simulink model "playground"  (R2024a)
settings: Solver=ode45  StartTime=0.0  StopTime=10.0  FixedStep=0.001  RelTol=1e-3
values from neighbouring files (symbols this model uses):
  a_r = 1.14 * 10^(-7)    (= 1.14e-07)    [start.m]    (also in startEnglPaper.m = 0.033; startReduced.m)
  a_rS = b    (= 0.033)    [startEnglPaper.m]
  A_x = 0.25    [playgrounMat.m]    (also in start.m; startEnglPaper.m; startReduced.m)
  A_y = 0.25    [playgrounMat.m]    (also in start.m; startEnglPaper.m; startReduced.m)
  A_z = 0.25    [playgrounMat.m]    (also in start.m; startEnglPaper.m; startReduced.m)
  b = 1.14 * 10^(-7)    (= 1.14e-07)    [start.m]    (also in startEnglPaper.m = 0.033; startReduced.m)
  g = 9.81    [playgrounMat.m]    (also in start.m; startEnglPaper.m; startReduced.m)
  gamma_d = pi/3    (= 1.0471975512)    [start.m]    (also in startReduced.m)
  I_r = 5.38 * 10 ^ (-5)    (= 5.38e-05)    [start.m]    (also in startEnglPaper.m = 3.38e-05; startReduced.m)
  I_x = 0.0151    [start.m]    (also in startEnglPaper.m = 0.004856; startReduced.m)
  I_y = 0.253    [start.m]    (also in startEnglPaper.m = 0.004856; startReduced.m)
  I_z = 0.0151    [start.m]    (also in startEnglPaper.m = 0.008801; startReduced.m)
  IrS = 5.38 * 10^(-5)    (= 5.38e-05)    [startEnglPaper.m]
  IxS = 0.0151    [startEnglPaper.m]
  IyS = IxS    (= 0.0151)    [startEnglPaper.m]
  IzS = 0.0253    [startEnglPaper.m]
  k = 1.045 * 10^(-11)    (= 1.045e-11)    [start.m]    (also in startEnglPaper.m = 2.98e-06; startReduced.m)
  K_gamma_D1 = K(1)    [playgrounMat.m]
  K_gamma_I1 = K(3)    [playgrounMat.m]
  K_gamma_P1 = K(2)    [playgrounMat.m]
  K_phi_D1 = 0.047    [startEnglPaper.m]
  K_phi_D11 = 0.093    [startEnglPaper.m]
  K_phi_D2 = 9.6    [startEnglPaper.m]
  K_phi_D22 = 19.2    [startEnglPaper.m]
  K_phi_DS = 0.14    [startEnglPaper.m]
  K_phi_I11 = 1.27    [startEnglPaper.m]
  K_phi_I22 = 262.144    [startEnglPaper.m]
  K_phi_P1 = 0.11    [startEnglPaper.m]
  K_phi_P11 = 0.5966    [startEnglPaper.m]
  K_phi_P2 = 23.04    [startEnglPaper.m]
  K_phi_P22 = 122.88    [startEnglPaper.m]
  K_phi_PS = 0.35    [startEnglPaper.m]
  K_psi_D = 40    [start.m]    (also in startEnglPaper.m = 9.6; startReduced.m)
  K_psi_D1 = 0.0844    [startEnglPaper.m]
  K_psi_D2 = 9.6    [startEnglPaper.m]
  K_psi_D22 = 19.2    [startEnglPaper.m]
  K_psi_DS = 0.24    [startEnglPaper.m]
  K_psi_I22 = 262.144    [startEnglPaper.m]
  K_psi_P = 143    [start.m]    (also in startEnglPaper.m = 23.04; startReduced.m)
  K_psi_P1 = 0.202    [startEnglPaper.m]
  K_psi_P2 = 23.04    [startEnglPaper.m]
  K_psi_P22 = 122.88    [startEnglPaper.m]
  K_psi_PS = 0.58    [startEnglPaper.m]
  K_theta_D = 58    [start.m]    (also in startEnglPaper.m = 9.6; startReduced.m)
  K_theta_D1 = 0.047    [startEnglPaper.m]
  K_theta_D2 = 9.6    [startEnglPaper.m]
  K_theta_D22 = 19.2    [startEnglPaper.m]
  K_theta_DS = 0.14    [startEnglPaper.m]
  K_theta_I22 = 262.144    [startEnglPaper.m]
  K_theta_P = 141    [start.m]    (also in startEnglPaper.m = 23.04; startReduced.m)
  K_theta_P1 = 0.11    [startEnglPaper.m]
  K_theta_P2 = 23.04    [startEnglPaper.m]
  K_theta_P22 = 122.88    [startEnglPaper.m]
  K_theta_PS = 0.35    [startEnglPaper.m]
  K_y_D = 13.58    [start.m]    (also in startReduced.m)
  K_y_P = 33.18    [start.m]    (also in startReduced.m)
  K_z_D1 = 4.42    [startEnglPaper.m]
  K_z_D2 = 4.42/m + A_z/m    (= 9.60905349794)    [startEnglPaper.m]
  K_z_DS = 13.58    [startEnglPaper.m]
  K_z_P1 = 11.2    [startEnglPaper.m]
  K_z_P2 = 11.2/m + A_z/m    (= 23.5596707819)    [startEnglPaper.m]
  K_z_PS = 33.18    [startEnglPaper.m]
  kl = 3 * 10^(-6)    (= 3e-06)    [startEnglPaper.m]
  l = 0.225    [start.m]    (also in startEnglPaper.m; startReduced.m)
  m = 1.44    [playgrounMat.m]    (also in start.m; startEnglPaper.m = 0.486; startReduced.m)
  m_s = [1/4 0 -1/(2*l) -1/(4*a_r); 1/4 -1/(2*l) 0 1/(4*a_r); 1/4 0 1/(2*l) -1/(4*a_r); 1/4 1/(2*l) 0 1/(4*a_r)]    [start.m]    (also in startReduced.m)
  mS = 1.44    [startEnglPaper.m]
  phi_d = 0.2    [startEnglPaper.m]
  phi_DesS = 0.2    [startEnglPaper.m]
  phi_init = 0    [startEnglPaper.m]
  phi_iS = 0;   deg2rad(10)    [startEnglPaper.m]
  psi_d = pi/5    (= 0.628318530718)    [start.m]    (also in startEnglPaper.m = 0.15; startReduced.m)
  psi_DesS = 0.15    [startEnglPaper.m]
  psi_init = 0    [startEnglPaper.m]
  psi_iS = 0    [startEnglPaper.m]
  theta_d = pi/4    (= 0.785398163397)    [start.m]    (also in startEnglPaper.m = 0.3; startReduced.m)
  theta_DesS = -0.1 * -3    (= 0.3)    [startEnglPaper.m]
  theta_init = 0    [startEnglPaper.m]
  theta_iS = 0    [startEnglPaper.m]
  x_init = 0    [startEnglPaper.m]
  x_iS = 0    [startEnglPaper.m]
  y_init = 0    [startEnglPaper.m]
  y_iS = 0    [startEnglPaper.m]
  z_d = 0.05 * 0    (= 0)    [startEnglPaper.m]
  z_DesS = 0.1    [startEnglPaper.m]
  z_init = 0    [startEnglPaper.m]
  z_iS = 0.0    (= 0)    [startEnglPaper.m]
undefined symbols (not defined in the file or in its folder): m_s_my
libraries: slpidlib x14
(part 4 of 4)

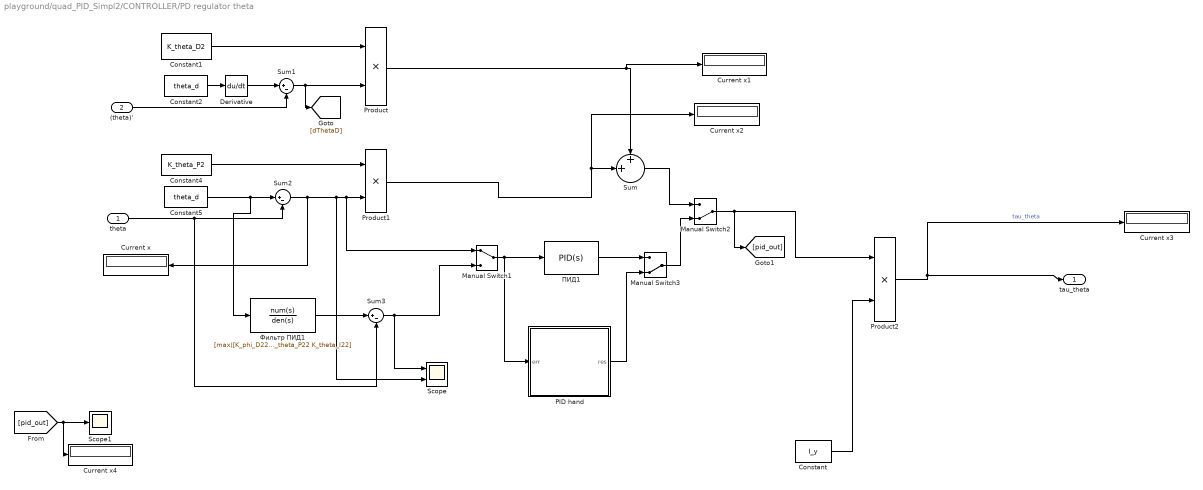
== system playground/quad_PID_Simpl2/CONTROLLER/PD regulator theta ==
  theta : Inport
  (theta)' : Inport  Port=2
  Constant : Constant  Value=I_y
  Constant1 : Constant  Value=K_theta_D2
  Constant2 : Constant  Value=theta_d
  Constant4 : Constant  Value=K_theta_P2
  Constant5 : Constant  Value=theta_d
  Current x{,1..4} (5 alike) : Display
  Derivative : Derivative
  Manual Switch1 : ManualSwitch
  Manual Switch2 : ManualSwitch  CurrentSetting=0
  Manual Switch3 : ManualSwitch  CurrentSetting=0
  PID hand : Subsystem
  Product : Product
  Product1 : Product
  Product2 : Product
  Scope : Scope  NumInputPorts=2
  Scope1 : Scope
  Sum : Sum  Inputs=++|
  Sum1 : Sum  Inputs=|+-
  Sum2 : Sum  Inputs=|+-
  Sum3 : Sum  Inputs=|+-
  ПИД1 : slpidlib/PID Controller  Controller=PID  Form=Parallel  TimeDomain=Continuous-time  UseExternalTs=off  SampleTime=-1  IntegratorMethod=Forward Euler  FilterMethod=Forward Euler  ControllerParametersSource=internal  P=K_theta_P22  I=K_theta_I22  UseKiTs=off  D=K_theta_D22  UseExternalDerivativeSource=off  N=1000  UseFilter=on  TunerSelectOption=Transfer Function Based (PID Tuner App)  InitialConditionSource=internal  InitialConditionForIntegrator=0  InitialConditionForFilter=0  DifferentiatorICPrevScaledInput=0  ExternalReset=none  TrackingMode=off  Kt=1  LimitOutput=on  SatLimitsSource=internal  UpperSaturationLimit=30  LowerSaturationLimit=-30  LinearizeAsGain=on  AntiWindupMode=none  Kb=1  LimitIntegrator=off  UpperIntegratorSaturationLimit=inf  LowerIntegratorSaturationLimit=-inf  POutMin=[]  POutMax=[]  IOutMin=[]  IOutMax=[]  DOutMin=[]  DOutMax=[]  NOutMin=[]  NOutMax=[]  SumOutMin=[]  SumOutMax=[]  SaturationOutMin=[]  SaturationOutMax=[]  PParamMin=[]  PParamMax=[]  IParamMin=[]  IParamMax=[]  DParamMin=[]  DParamMax=[]  NParamMin=[]  NParamMax=[]  KbParamMin=[]  KbParamMax=[]  KtParamMin=[]  KtParamMax=[]  KbOutMin=[]  KbOutMax=[]  KtOutMin=[]  KtOutMax=[]  IntegratorOutMin=[]  IntegratorOutMax=[]  FilterOutMin=[]  FilterOutMax=[]  SumI1OutMin=[]  SumI1OutMax=[]  SumI2OutMin=[]  SumI2OutMax=[]  SumI3OutMin=[]  SumI3OutMax=[]  SumI4OutMin=[]  SumI4OutMax=[]  SumDOutMin=[]  SumDOutMax=[]  DifferentiatorOutMin=[]  DifferentiatorOutMax=[]  FilterDiffOutCoefMin=[]  FilterDiffOutCoefMax=[]  ReciprocalOutMin=[]  ReciprocalOutMax=[]  SumDenOutMin=[]  SumDenOutMax=[]  SumNumOutMin=[]  SumNumOutMax=[]  DivideOutMin=[]  DivideOutMax=[]  UdiffTsProdOutMin=[]  UdiffTsProdOutMax=[]  NTsProdOutMin=[]  NTsProdOutMax=[]  UintegralTsProdOutMin=[]  UintegralTsProdOutMax=[]  UngainTsProdOutMin=[]  UngainTsProdOutMax=[]  ClampingZeroOutDataTypeStr=Inherit: Inherit via back propagation  ClampingZeroOutMin=[]  ClampingZeroOutMax=[]  FilterDenConstantOutDataTypeStr=Inherit: Inherit via back propagation  FilterDenConstantOutMin=[]  FilterDenConstantOutMax=[]  PCopyOutDataTypeStr=Inherit: Inherit via back propagation  PCopyOutMin=[]  PCopyOutMax=[]  NCopyOutDataTypeStr=Inherit: Inherit via back propagation  NCopyOutMin=[]  NCopyOutMax=[]  IntegratorContinuousStateAttributes=''  IntegratorStateMustResolveToSignalObject=off  IntegratorRTWStateStorageClass=Auto  FilterContinuousStateAttributes=''  FilterStateMustResolveToSignalObject=off  FilterRTWStateStorageClass=Auto  ParallelPVariant=InternalParameters  IdealPVariant=Disabled  IVariant=InternalParameters  DVariant=InternalParameters  IntegratorVariant=Continuous  SatVariant=Enabled  AWVariant=Passthrough  PCopyVariant=Disabled  TRVariant=Disabled  FdbkBlocksVariant=Forward  IdealPFdbkVariant=Disabled  SatFdbkVariant=Disabled  DerivativeFilterVariant=ContFilter  NVariant=InternalParameters  NCopyVariant=Disabled  FilterICVariant=InternalICsFilter  IntegratorICVariant=InternalICs  ExternalResetVariant=Disabled  TRSumVariant=Passthrough  SumFdbkVariant=Disabled  SumVariant=Sum_PID  TsampFilterVariant=InternalTs  TsampNgainVariant=Passthrough  TsampIntegralVariant=Disabled_SignalSpec  ExternalSaturationOutDataTypeStr=Inherit: Same as second input  DerivativeSourceVariant=ErrorSignal
  Фильтр ПИД1 : TransferFcn  Numerator=[max([K_phi_D22 K_phi_P22 K_phi_I22])]  Denominator=[K_theta_D22 K_theta_P22 K_theta_I22]
  tau_theta : Outport
  wires:
  Constant/1 -> Product2/2
  Product2/1 -> Current x3/1, tau_theta/1  "tau_theta"
  Sum2/1 -> Scope/2, Manual Switch1/1, Product1/2, Current x/1
  (theta)'/1 -> Sum1/2
  Constant2/1 -> Derivative/1
  Derivative/1 -> Sum1/1
  Constant5/1 -> Фильтр ПИД1/1, Sum2/1
  theta/1 -> Sum2/2, Sum3/2
  Constant4/1 -> Product1/1
  Sum1/1 -> [dThetaD], Product/2
  Product1/1 -> Current x2/1, Sum/2
  Constant1/1 -> Product/1
  Product/1 -> Sum/1, Current x1/1
  Sum/1 -> Manual Switch2/1
  Manual Switch1/1 -> ПИД1/1, PID hand/1(err)
  Manual Switch2/1 -> [pid_out], Product2/1
  Фильтр ПИД1/1 -> Sum3/1
  Sum3/1 -> Scope/1, Manual Switch1/2
  Manual Switch3/1 -> Manual Switch2/2
  PID hand/1(res) -> Manual Switch3/2
  [pid_out] -> Current x4/1, Scope1/1
  ПИД1/1 -> Manual Switch3/1

== system playground/ST_constants_useIX/CONTROLLER/PD regulator gamma1/PID hand ==
  err : Inport
  Derivative1 : Derivative
  Gain1 : Gain  Gain=K_phi_P22
  Gain2 : Gain  Gain=K_phi_D22
  Gain3 : Gain  Gain=K_phi_I22
  Integrator1 : Integrator
  Manual Switch : ManualSwitch
  Saturation : Saturate  UpperLimit=20  LowerLimit=-20
  Scope : Scope
  Scope1 : Scope
  Scope8 : Scope  NumInputPorts=3
  Sum : Sum  Inputs=|+++
  res : Outport
  wires:
  Derivative1/1 -> Gain2/1
  Integrator1/1 -> Gain3/1
  err/1 -> Scope1/1, Derivative1/1, Gain1/1, Integrator1/1
  Gain2/1 -> [D_out]
  Gain3/1 -> [I_out]
  Gain1/1 -> [P_out]
  [I_out] -> Scope8/1  "I"
  [P_out] -> Scope8/2  "P"
  [D_out] -> Scope8/3  "D"
  [D_out] -> Sum/1
  [I_out] -> Sum/2
  [P_out] -> Sum/3
  Sum/1 -> Saturation/1, Manual Switch/2, Scope/1
  Saturation/1 -> Manual Switch/1
  Manual Switch/1 -> res/1

== system playground/quad_PID_Simpl2/CONTROLLER/PD regulator gamma1/PID hand ==
  err : Inport
  Derivative1 : Derivative
  Gain1 : Gain  Gain=K_phi_P22
  Gain2 : Gain  Gain=K_phi_D22
  Gain3 : Gain  Gain=K_phi_I22
  Integrator1 : Integrator
  Manual Switch : ManualSwitch
  Saturation : Saturate  UpperLimit=20  LowerLimit=-20
  Scope : Scope
  Scope1 : Scope
  Scope8 : Scope  NumInputPorts=3
  Sum : Sum  Inputs=|+++
  res : Outport
  wires:
  Derivative1/1 -> Gain2/1
  Integrator1/1 -> Gain3/1
  err/1 -> Scope1/1, Derivative1/1, Gain1/1, Integrator1/1
  Gain2/1 -> [D_out]
  Gain3/1 -> [I_out]
  Gain1/1 -> [P_out]
  [I_out] -> Scope8/1  "I"
  [P_out] -> Scope8/2  "P"
  [D_out] -> Scope8/3  "D"
  [D_out] -> Sum/1
  [I_out] -> Sum/2
  [P_out] -> Sum/3
  Sum/1 -> Saturation/1, Manual Switch/2, Scope/1
  Saturation/1 -> Manual Switch/1
  Manual Switch/1 -> res/1

== system playground/quad_PID_Simpl2/CONTROLLER/PD regulator psi/PID hand ==
  err : Inport
  Derivative1 : Derivative
  Gain1 : Gain  Gain=K_psi_P22
  Gain2 : Gain  Gain=K_psi_D22
  Gain3 : Gain  Gain=K_psi_I22
  Integrator1 : Integrator
  Manual Switch : ManualSwitch
  SAT : Saturate  UpperLimit=10  LowerLimit=-5
  Scope : Scope
  Scope1 : Scope
  Scope8 : Scope  NumInputPorts=3
  Sum : Sum  Inputs=|+++
  res : Outport
  wires:
  Derivative1/1 -> Gain2/1
  Integrator1/1 -> Gain3/1
  err/1 -> Derivative1/1, Gain1/1, Integrator1/1
  Gain2/1 -> [D_out]
  Gain3/1 -> [I_out]
  Gain1/1 -> [P_out]
  [I_out] -> Scope8/1  "I"
  [P_out] -> Scope8/2  "P"
  [D_out] -> Scope8/3  "D"
  [D_out] -> Sum/1
  [I_out] -> Sum/2
  [P_out] -> Sum/3
  Sum/1 -> SAT/1, Scope/1, Manual Switch/2
  SAT/1 -> Scope1/1, Manual Switch/1
  Manual Switch/1 -> res/1

== system playground/quad_PID_Simpl2/CONTROLLER/PD regulator theta/PID hand ==
  err : Inport
  Derivative2 : Derivative
  Gain1 : Gain  Gain=K_theta_P22
  Gain2 : Gain  Gain=K_theta_D22
  Gain3 : Gain  Gain=K_theta_I22
  Integrator2 : Integrator
  Manual Switch : ManualSwitch
  Saturation : Saturate  UpperLimit=30  LowerLimit=-30
  Scope : Scope
  Scope1 : Scope
  Scope8 : Scope  NumInputPorts=3
  Sum : Sum  Inputs=|+++
  res : Outport
  wires:
  err/1 -> Scope1/1, Gain3/1, Gain2/1, Gain1/1
  Gain2/1 -> Derivative2/1
  Gain3/1 -> Integrator2/1
  Gain1/1 -> [P_out]
  [I_out] -> Scope8/1  "I"
  [P_out] -> Scope8/2  "P"
  [D_out] -> Scope8/3  "D"
  [D_out] -> Sum/1
  [I_out] -> Sum/2
  [P_out] -> Sum/3
  Integrator2/1 -> [I_out]
  Derivative2/1 -> [D_out]
  Manual Switch/1 -> res/1
  Sum/1 -> Manual Switch/2, Saturation/1, Scope/1
  Saturation/1 -> Manual Switch/1

== matlab function playground/ST_constants_no_IX/CONTROLLER/PD regulator draft/m//cos(y)*(cos(theta)) ==
  data: m input; c output; phi input; theta input
function c = fcn(m, phi, theta)

c = m / (cos(phi)*cos(theta));

== matlab function playground/ST_constants_no_IX/OMEGA_2_TAU/Gyroscope ==
  data: w_1 input; w_2 input; w_3 input; w_Gamma output; w_4 input
function w_Gamma = fcn(w_1, w_2, w_3, w_4)
    
w_Gamma = w_1 - w_2 + w_3 - w_4;

== matlab function playground/ST_constants_no_IX/OMEGA_2_TAU/MATLAB Function ==
  data: w1 input; T output; w2 input; w3 input; w4 input; k input
function T = fcn(w1, w2, w3, w4, k)

T = k*(w1^2 + w2^2 + w3^2 + w4^2);

== matlab function playground/ST_constants_no_IX/OMEGA_2_TAU/MATLAB Function1 ==
  data: w2 input; tau_phi output; w4 input; kl input
function tau_phi = fcn(w2, w4, kl)

tau_phi = kl*(-w2^2 + w4^2);

== matlab function playground/ST_constants_no_IX/OMEGA_2_TAU/MATLAB Function2 ==
  data: w1 input; tau_theta output; w3 input; kl input
function tau_theta = fcn(w1, w3, kl)

tau_theta = kl* (-w1^2 + w3^2);

== matlab function playground/ST_constants_no_IX/OMEGA_2_TAU/MATLAB Function3 ==
  data: w1 input; tau_psi output; w2 input; w3 input; w4 input; b input
function tau_psi = fcn(w1, w2, w3, w4, b)

tau_psi = b * (-w1^2 + w2^2 - w3^2 + w4^2);
%tau_psi = b * (w1 - w2 + w3 - w4);

== matlab function playground/ST_constants_no_IX/TAU_2_OMEGA/MATLAB Function1 ==
  data: T input; omega_1 output; omega_2 output; omega_3 output; omega_4 output; tau_phi input; tau_theta input; tau_psi input; k input; l input; b input
function [omega_1,omega_2,omega_3,omega_4] = fcn(T,tau_phi,tau_theta,tau_psi,k,l,b)
%omega_1 = tau_y/(4*k) + tau_theta/(2*k*l) + tau_psi/(4*b);
%omega_2 = tau_y/(4*k) + tau_gamma/(2*k*l) - tau_psi/(4*b);
%omega_3 = tau_y/(4*k) - tau_theta/(2*k*l) + tau_psi/(4*b);  % измененные по решению системы уравнений
%omega_4 = tau_y/(4*k) - tau_gamma/(2*k*l) - tau_psi/(4*b);

omega_1 = T/(4*k) - tau_theta/(2*k*l) - tau_psi/(4*b);
omega_2 = T/(4*k) - tau_phi/(2*k*l) + tau_psi/(4*b);  % согласно статье
omega_3 = T/(4*k) + tau_theta/(2*k*l) - tau_psi/(4*b);
omega_4 = T/(4*k) + tau_phi/(2*k*l) + tau_psi/(4*b);

== matlab function playground/ST_constants_no_IX/XYZ POSITION/XYZ ==
  data: T input; ddx output; m input; Ax input; Ay input; Az input; phi input; theta input; psi input; dx input; dy input; dz input; ddy output; ddz output
function [ddx, ddy, ddz] = fcn(T, m, Ax, Ay, Az, phi, theta, psi, dx, dy, dz)

g = 9.81;

ddx = (T/m)*(cos(psi)*sin(theta)*cos(phi) + sin(psi)*sin(phi)) - Ax*dx/m;
ddy = (T/m)*(sin(psi)*sin(theta)*cos(phi) - cos(psi)*sin(phi)) - Ay*dy/m;

ddz = -g + (T/m)*(cos(theta)*cos(phi)) - Az*dz/m;

== matlab function playground/ST_constants_useIX/ANGLE VELOCITY PQR(wx,xy,xz)/p_part ==
  data: Ix input; Iy input; dp output; Iz input; Ir input; q input; r input; wr input; tau_phi input
function dp = fcn(Ix, Iy, Iz, Ir, q, r,  wr, tau_phi)

dp = (Iy - Iz)*q*r/Ix - Ir*q*wr/Ix + tau_phi/Ix;
%dp =  tau_phi/Ix;

== matlab function playground/ST_constants_no_IX/ANGLE VELOCITY PQR(wx,xy,xz)/p_part ==
  data: Ix input; Iy input; dp output; Iz input; Ir input; q input; r input; wr input; tau_phi input
function dp = fcn(Ix, Iy, Iz, Ir, q, r,  wr, tau_phi)

dp = (Iy - Iz)*q*r/Ix - Ir*q*wr/Ix + tau_phi/Ix;
%dp =  tau_phi/Ix;

== matlab function playground/quad_PID_Simpl/9_form_omega/omega_y' ==
  data: I_z input; I_x input; I_y input; domega_y output; omega_x input; omega_z input; tau_psi input
function domega_y = fcn(I_z, I_x, I_y, omega_x, omega_z, tau_psi)

tmp = (I_z - I_x)*omega_x*omega_z + tau_psi;
domega_y = tmp / I_y;

== matlab function playground/quad_PID_Simpl/9_form_omega/omega_z' ==
  data: I_y input; domega_z output; I_x input; I_z input; I_r input; omega_y input; omega_x input; omega_r input; tau_theta input
function domega_z = fcn(I_y, I_x, I_z, I_r, omega_y, omega_x, omega_r, tau_theta)

tmp = (I_x - I_y)*omega_x*omega_y + I_r*omega_x*omega_r + tau_theta;


domega_z = tmp / I_z;

== matlab function playground/quad_PID_Simpl/Angle_moving/MFgamma ==
  data: omega_x input; d_gamma output; omega_y input; omega_z input; gamma input; theta input
function d_gamma = fcn(omega_x, omega_y, omega_z, gamma, theta)

d_gamma = omega_x + sin(gamma)*tan(theta)*omega_z + cos(gamma)*tan(theta)*omega_y;

== matlab function playground/quad_PID_Simpl/Angle_moving/MFpsi ==
  data: d_psi output; omega_y input; omega_z input; gamma input; theta input
function d_psi = fcn(omega_y, omega_z, gamma, theta)

d_psi = sin(gamma)*omega_z/cos(theta) + cos(gamma)*omega_y/cos(theta);

== matlab function playground/quad_PID_Simpl/Angle_moving/MFtheta ==
  data: d_theta output; omega_y input; omega_z input; gamma input
function d_theta = fcn(omega_y, omega_z, gamma)

d_theta = cos(gamma)*omega_z - sin(gamma)*omega_y;

== matlab function playground/quad_PID_Simpl/Form6_w ==
  data: kl input; l input; a_r input; tau_y1 output; w1 input; w2 input; w3 input; w4 input; tau_gamma1 output; tau_theta1 output; tau_psi1 output; w_R output
function [tau_y1, tau_gamma1, tau_theta1, tau_psi1, w_R] = fcn(kl, l, a_r, w1, w2, w3, w4)
tau_y1 = kl*(w1+w2+w3+w4);
tau_gamma1 = kl*l*(w2-w4);
tau_theta1 = kl*l*(w1-w3);
tau_psi1 = a_r*(w1-w2+w3-w4); %a_r
w_R = w1-w2+w3-w4;

== matlab function playground/quad_PID_Simpl/MATLAB Function ==
  data: tau_y input; omega_1 output; omega_2 output; omega_3 output; omega_4 output; tau_gamma input; tau_theta input; tau_psi input; k input; l input; b input
function [omega_1,omega_2,omega_3,omega_4] = fcn(tau_y,tau_gamma,tau_theta,tau_psi,k,l,b)
omega_1 = tau_y/(4*k) - tau_theta/(2*k*l) - tau_psi/(4*b);
omega_2 = tau_y/(4*k) - tau_gamma/(2*k*l) + tau_psi/(4*b);
omega_3 = tau_y/(4*k) + tau_theta/(2*k*l) - tau_psi/(4*b);
omega_4 = tau_y/(4*k) + tau_gamma/(2*k*l) + tau_psi/(4*b);

== matlab function playground/quad_PID_Simpl/MATLAB Function2 ==
  data: tau_arr input; w1 output; M input; w2 output; w3 output; w4 output; w1234 output
function [w1,w2,w3,w4, w1234] = fcn(tau_arr, M)
w1234 = M * [tau_arr(1);tau_arr(2);tau_arr(3);tau_arr(4)];
w1 = w1234(1);
w2 = w1234(2);
w3 = w1234(3);
w4 = w1234(4);

== matlab function playground/quad_PID_Simpl/PD regulator draft/m//cos(y)*(cos(theta)) ==
  data: m input; c output; gamma input; theta input
function c = fcn(m, gamma, theta)

c = m / (cos(gamma)*cos(theta));

== matlab function playground/quad_PID_Simpl/TAU_SAT ==
  data: kl input; l input; a_r input; tau_y1 output; w1 input; w2 input; w3 input; w4 input; tau_gamma1 output; tau_theta1 output; tau_psi1 output; w_R output
function [tau_y1, tau_gamma1, tau_theta1, tau_psi1, w_R] = fcn(kl, l, a_r, w1, w2, w3, w4)
tau_y1 = kl*(w1+w2+w3+w4);
tau_gamma1 = kl*l*(w2-w4);
tau_theta1 = kl*l*(w1-w3);
tau_psi1 = a_r*(w1-w2+w3-w4);
w_R = w1-w2+w3-w4;

== matlab function playground/quad_PID_Simpl/MATLAB Function1 ==
  data: tau_y input; omega_1 output; omega_2 output; omega_3 output; omega_4 output; tau_gamma input; tau_theta input; tau_psi input; k input; l input; b input
function [omega_1,omega_2,omega_3,omega_4] = fcn(tau_y,tau_gamma,tau_theta,tau_psi,k,l,b)
omega_1 = tau_y/(4*k) + tau_theta/(2*k*l) + tau_psi/(4*b);
omega_2 = tau_y/(4*k) + tau_gamma/(2*k*l) - tau_psi/(4*b);
omega_3 = tau_y/(4*k) - tau_theta/(2*k*l) + tau_psi/(4*b);  % измененные по решению системы уравнений
omega_4 = tau_y/(4*k) - tau_gamma/(2*k*l) - tau_psi/(4*b);

%omega_1 = tau_y/(4*k) - tau_theta/(2*k*l) - tau_psi/(4*b);
%omega_2 = tau_y/(4*k) - tau_gamma/(2*k*l) + tau_psi/(4*b);  % согласно статье
%omega_3 = tau_y/(4*k) + tau_theta/(2*k*l) - tau_psi/(4*b);
%omega_4 = tau_y/(4*k) + tau_gamma/(2*k*l) + tau_psi/(4*b);

== matlab function playground/ST_constants_no_IX/ANGLE VELOCITY PQR(wx,xy,xz)/q_part ==
  data: Ix input; Iy input; dq output; Iz input; Ir input; wr input; p input; r input; tau_theta input
function dq = fcn(Ix, Iy, Iz, Ir, wr, p, r, tau_theta)

dq = (Iz - Ix)*p*r/Iy + Ir*p*wr/Iy + tau_theta/Iy;

== matlab function playground/quad_PID_Simpl/Form6_w1 ==
  data: kl input; l input; a_r input; tau_y1 output; w input; tau_gamma1 output; tau_theta1 output; tau_psi1 output; w_R output
function [tau_y1, tau_gamma1, tau_theta1, tau_psi1, w_R] = fcn(kl, l, a_r, w)

w1 = w(1);
w2 = w(2);
w3 = w(3);
w4 = w(4);

tau_y1 = kl*(w1+w2+w3+w4);
tau_gamma1 = kl*l*(w2-w4);
tau_theta1 = kl*l*(w1-w3);
tau_psi1 = a_r*(w1-w2+w3-w4); %a_r
w_R = sqrt(w1)-sqrt(w2)+sqrt(w3)-sqrt(w4);
%w_R = w1 - w2 + w3 - w4;

== matlab function playground/CHANGE_PID/ANGLE VELOCITY PQR(wx,xy,xz)/p_part ==
  data: Ix input; Iy input; dp output; Iz input; Ir input; q input; r input; wr input; tau_phi input
function dp = fcn(Ix, Iy, Iz, Ir, q, r,  wr, tau_phi)

dp = (Iy - Iz)*q*r/Ix - Ir*q*wr/Ix + tau_phi/Ix;

== matlab function playground/CHANGE_PID/ANGLE VELOCITY PQR(wx,xy,xz)/q_part ==
  data: Ix input; Iy input; dq output; Iz input; Ir input; wr input; p input; r input; tau_theta input
function dq = fcn(Ix, Iy, Iz, Ir, wr, p, r, tau_theta)

dq = (Iz - Ix)*p*r/Iy + Ir*p*wr/Iy + tau_theta/Iy;

== matlab function playground/CHANGE_PID/ANGLE VELOCITY PQR(wx,xy,xz)/r_part ==
  data: Ix input; dr output; Iy input; Iz input; p input; q input; tau_psi input
function dr = fcn(Ix, Iy, Iz, p, q, tau_psi)

dr = (Ix - Iy)*p*q/Iz + tau_psi/Iz;

== matlab function playground/CHANGE_PID/ANGLS/phi_part ==
  data: p input; d_phi output; q input; r input; phi input; theta input
function d_phi = fcn(p,q,r, phi, theta)

d_phi = p + sin(phi)*cos(theta)*q + cos(phi)*tan(theta)*r;

== matlab function playground/CHANGE_PID/ANGLS/psi_part ==
  data: q input; d_psi output; r input; phi input; theta input
function d_psi = fcn(q, r, phi, theta)

d_psi = q*sin(phi)/cos(theta) + r*cos(phi)/cos(theta);

== matlab function playground/CHANGE_PID/ANGLS/theta_part ==
  data: q input; d_theta output; r input; phi input
function d_theta = fcn(q, r, phi)

d_theta = cos(phi)*q - sin(phi)*r;

== matlab function playground/CHANGE_PID/CONTROLLER/PD regulator draft/m//cos(y)*(cos(theta)) ==
  data: m input; c output; phi input; theta input
function c = fcn(m, phi, theta)

c = m / (cos(phi)*cos(theta));

== matlab function playground/CHANGE_PID/OMEGA_2_TAU/Gyroscope ==
  data: w_1 input; w_2 input; w_3 input; w_Gamma output; w_4 input
function w_Gamma = fcn(w_1, w_2, w_3, w_4)
    
w_Gamma = w_1 - w_2 + w_3 - w_4;

== matlab function playground/CHANGE_PID/OMEGA_2_TAU/MATLAB Function ==
  data: w1 input; T output; w2 input; w3 input; w4 input; k input
function T = fcn(w1, w2, w3, w4, k)

T = k*(w1^2 + w2^2 + w3^2 + w4^2);

== matlab function playground/CHANGE_PID/OMEGA_2_TAU/MATLAB Function1 ==
  data: w2 input; tau_phi output; w4 input; kl input
function tau_phi = fcn(w2, w4, kl)

tau_phi = kl*(-w2^2 + w4^2);

== matlab function playground/CHANGE_PID/OMEGA_2_TAU/MATLAB Function2 ==
  data: w1 input; tau_theta output; w3 input; kl input
function tau_theta = fcn(w1, w3, kl)

tau_theta = kl* (-w1^2 + w3^2);

== matlab function playground/ST_constants_no_IX/ANGLE VELOCITY PQR(wx,xy,xz)/r_part ==
  data: Ix input; dr output; Iy input; Iz input; p input; q input; tau_psi input
function dr = fcn(Ix, Iy, Iz, p, q, tau_psi)

dr = (Ix - Iy)*p*q/Iz + tau_psi/Iz;

== matlab function playground/CHANGE_PID/OMEGA_2_TAU/MATLAB Function3 ==
  data: w1 input; tau_psi output; w2 input; w3 input; w4 input; b input
function tau_psi = fcn(w1, w2, w3, w4, b)

tau_psi = b * (-w1^2 + w2^2 - w3^2 + w4^2);

== matlab function playground/CHANGE_PID/TAU_2_OMEGA/MATLAB Function1 ==
  data: T input; omega_1 output; omega_2 output; omega_3 output; omega_4 output; tau_phi input; tau_theta input; tau_psi input; k input; l input; b input
function [omega_1,omega_2,omega_3,omega_4] = fcn(T,tau_phi,tau_theta,tau_psi,k,l,b)
%omega_1 = tau_y/(4*k) + tau_theta/(2*k*l) + tau_psi/(4*b);
%omega_2 = tau_y/(4*k) + tau_gamma/(2*k*l) - tau_psi/(4*b);
%omega_3 = tau_y/(4*k) - tau_theta/(2*k*l) + tau_psi/(4*b);  % измененные по решению системы уравнений
%omega_4 = tau_y/(4*k) - tau_gamma/(2*k*l) - tau_psi/(4*b);

omega_1 = T/(4*k) - tau_theta/(2*k*l) - tau_psi/(4*b);
omega_2 = T/(4*k) - tau_phi/(2*k*l) + tau_psi/(4*b);  % согласно статье
omega_3 = T/(4*k) + tau_theta/(2*k*l) - tau_psi/(4*b);
omega_4 = T/(4*k) + tau_phi/(2*k*l) + tau_psi/(4*b);

== matlab function playground/CHANGE_PID/XYZ POSITION/XYZ ==
  data: T input; ddx output; m input; Ax input; Ay input; Az input; phi input; theta input; psi input; dx input; dy input; dz input; ddy output; ddz output
function [ddx, ddy, ddz] = fcn(T, m, Ax, Ay, Az, phi, theta, psi, dx, dy, dz)

g = 9.81;

ddx = (T/m)*(cos(psi)*sin(theta)*cos(phi) + sin(psi)*sin(phi)) - Ax*dx/m;
ddy = (T/m)*(sin(psi)*sin(theta)*cos(phi) - cos(psi)*sin(phi)) - Ay*dy/m;

ddz = -g + (T/m)*(cos(theta)*cos(phi)) - Az*dz/m;

== matlab function playground/ST_constants_useIX/ANGLE VELOCITY PQR(wx,xy,xz)/q_part ==
  data: Ix input; Iy input; dq output; Iz input; Ir input; wr input; p input; r input; tau_theta input
function dq = fcn(Ix, Iy, Iz, Ir, wr, p, r, tau_theta)

dq = (Iz - Ix)*p*r/Iy + Ir*p*wr/Iy + tau_theta/Iy;

== matlab function playground/quad_PID_Simpl2/CONTROLLER/PD regulator draft/m//cos(y)*(cos(theta)) ==
  data: m input; c output; phi input; theta input
function c = fcn(m, phi, theta)

c = m / (cos(phi)*cos(theta));

== matlab function playground/quad_PID_Simpl2/TAU_2_OMEGA/MATLAB Function1 ==
  data: T input; omega_1 output; omega_2 output; omega_3 output; omega_4 output; tau_phi input; tau_theta input; tau_psi input; k input; l input; b input
function [omega_1,omega_2,omega_3,omega_4] = fcn(T,tau_phi,tau_theta,tau_psi,k,l,b)
%omega_1 = tau_y/(4*k) + tau_theta/(2*k*l) + tau_psi/(4*b);
%omega_2 = tau_y/(4*k) + tau_gamma/(2*k*l) - tau_psi/(4*b);
%omega_3 = tau_y/(4*k) - tau_theta/(2*k*l) + tau_psi/(4*b);  % измененные по решению системы уравнений
%omega_4 = tau_y/(4*k) - tau_gamma/(2*k*l) - tau_psi/(4*b);

omega_1 = T/(4*k) - tau_theta/(2*k*l) - tau_psi/(4*b);
omega_2 = T/(4*k) - tau_phi/(2*k*l) + tau_psi/(4*b);  % согласно статье
omega_3 = T/(4*k) + tau_theta/(2*k*l) - tau_psi/(4*b);
omega_4 = T/(4*k) + tau_phi/(2*k*l) + tau_psi/(4*b);

== matlab function playground/quad_PID_Simpl2/OMEGA_2_TAU/MATLAB Function ==
  data: w1 input; T output; w2 input; w3 input; w4 input; k input
function T = fcn(w1, w2, w3, w4, k)

T = k*(w1^2 + w2^2 + w3^2 + w4^2);

== matlab function playground/quad_PID_Simpl2/OMEGA_2_TAU/MATLAB Function1 ==
  data: w2 input; tau_phi output; w4 input; kl input
function tau_phi = fcn(w2, w4, kl)

tau_phi = kl*(-w2^2 + w4^2);

== matlab function playground/quad_PID_Simpl2/OMEGA_2_TAU/MATLAB Function2 ==
  data: w1 input; tau_theta output; w3 input; kl input
function tau_theta = fcn(w1, w3, kl)

tau_theta = kl* (-w1^2 + w3^2);

== matlab function playground/ST_constants_no_IX/ANGLS/phi_part ==
  data: p input; d_phi output; q input; r input; phi input; theta input
function d_phi = fcn(p,q,r, phi, theta)

d_phi = p + sin(phi)*cos(theta)*q + cos(phi)*tan(theta)*r;
%d_phi = p;

== matlab function playground/quad_PID_Simpl2/OMEGA_2_TAU/MATLAB Function3 ==
  data: w1 input; tau_psi output; w2 input; w3 input; w4 input; b input; err output
function [tau_psi, err] = fcn(w1, w2, w3, w4, b)

tau_psi = b * (-w1^2 + w2^2 - w3^2 + w4^2);
err = -w1^2 + w2^2 - w3^2 + w4^2;

== matlab function playground/quad_PID_Simpl2/OMEGA_2_TAU/Gyroscope ==
  data: w_1 input; w_2 input; w_3 input; w_Gamma output; w_4 input
function w_Gamma = fcn(w_1, w_2, w_3, w_4)
    
w_Gamma = w_1 - w_2 + w_3 - w_4;

== matlab function playground/quad_PID_Simpl2/ANGLE VELOCITY PQR(wx,xy,xz)/p_part ==
  data: Ix input; Iy input; dp output; Iz input; Ir input; q input; r input; wr input; tau_phi input
function dp = fcn(Ix, Iy, Iz, Ir, q, r,  wr, tau_phi)

dp = (Iy - Iz)*q*r/Ix - Ir*q*wr/Ix + tau_phi/Ix;
%dp =  tau_phi/Ix;

== matlab function playground/quad_PID_Simpl2/ANGLE VELOCITY PQR(wx,xy,xz)/q_part ==
  data: Ix input; Iy input; dq output; Iz input; Ir input; wr input; p input; r input; tau_theta input
function dq = fcn(Ix, Iy, Iz, Ir, wr, p, r, tau_theta)

dq = (Iz - Ix)*p*r/Iy + Ir*p*wr/Iy + tau_theta/Iy;

== matlab function playground/quad_PID_Simpl2/ANGLE VELOCITY PQR(wx,xy,xz)/r_part ==
  data: Ix input; dr output; Iy input; Iz input; p input; q input; tau_psi input
function dr = fcn(Ix, Iy, Iz, p, q, tau_psi)

dr = (Ix - Iy)*p*q/Iz + tau_psi/Iz;

== matlab function playground/quad_PID_Simpl2/ANGLS/phi_part ==
  data: p input; d_phi output; q input; r input; phi input; theta input
function d_phi = fcn(p,q,r, phi, theta)

d_phi = p + sin(phi)*cos(theta)*q + cos(phi)*tan(theta)*r;
%d_phi = p;

== matlab function playground/quad_PID_Simpl2/ANGLS/theta_part ==
  data: q input; d_theta output; r input; phi input
function d_theta = fcn(q, r, phi)

d_theta = cos(phi)*q - sin(phi)*r;

== matlab function playground/quad_PID_Simpl2/ANGLS/psi_part ==
  data: q input; d_psi output; r input; phi input; theta input
function d_psi = fcn(q, r, phi, theta)

d_psi = q*sin(phi)/cos(theta) + r*cos(phi)/cos(theta);

== matlab function playground/quad_PID_Simpl2/XYZ POSITION/XYZ ==
  data: T input; ddx output; m input; Ax input; Ay input; Az input; phi input; theta input; psi input; dx input; dy input; dz input; ddy output; ddz output
function [ddx, ddy, ddz] = fcn(T, m, Ax, Ay, Az, phi, theta, psi, dx, dy, dz)

g = 9.81;

ddx = (T/m)*(cos(psi)*sin(theta)*cos(phi) + sin(psi)*sin(phi)) - Ax*dx/m;
ddy = (T/m)*(sin(psi)*sin(theta)*cos(phi) - cos(psi)*sin(phi)) - Ay*dy/m;

ddz = -g + (T/m)*(cos(theta)*cos(phi)) - Az*dz/m;

== matlab function playground/quad_PID_Simpl/9_form_omega/omega_x' ==
  data: I_y input; domega_x output; I_x input; I_z input; I_r input; omega_y input; omega_z input; omega_r input; tau_gamma input
function domega_x = fcn(I_y, I_x, I_z, I_r, omega_y, omega_z, omega_r, tau_gamma)

tmp = (I_y - I_z)*omega_y*omega_z - I_r*omega_z*omega_r + tau_gamma;

domega_x = tmp / I_x;

== matlab function playground/ST_constants_useIX/ANGLE VELOCITY PQR(wx,xy,xz)/r_part ==
  data: Ix input; dr output; Iy input; Iz input; p input; q input; tau_psi input
function dr = fcn(Ix, Iy, Iz, p, q, tau_psi)

dr = (Ix - Iy)*p*q/Iz + tau_psi/Iz;

== matlab function playground/ST_constants_useIX/ANGLS/phi_part ==
  data: p input; d_phi output; q input; r input; phi input; theta input
function d_phi = fcn(p,q,r, phi, theta)

d_phi = p + sin(phi)*cos(theta)*q + cos(phi)*tan(theta)*r;
%d_phi = p;

== matlab function playground/ST_constants_useIX/ANGLS/psi_part ==
  data: q input; d_psi output; r input; phi input; theta input
function d_psi = fcn(q, r, phi, theta)

d_psi = q*sin(phi)/cos(theta) + r*cos(phi)/cos(theta);

== matlab function playground/ST_constants_useIX/ANGLS/theta_part ==
  data: q input; d_theta output; r input; phi input
function d_theta = fcn(q, r, phi)

d_theta = cos(phi)*q - sin(phi)*r;

== matlab function playground/ST_constants_useIX/CONTROLLER/PD regulator draft/m//cos(y)*(cos(theta)) ==
  data: m input; c output; phi input; theta input
function c = fcn(m, phi, theta)

c = m / (cos(phi)*cos(theta));

== matlab function playground/ST_constants_useIX/OMEGA_2_TAU/Gyroscope ==
  data: w_1 input; w_2 input; w_3 input; w_Gamma output; w_4 input
function w_Gamma = fcn(w_1, w_2, w_3, w_4)
    
w_Gamma = w_1 - w_2 + w_3 - w_4;

== matlab function playground/ST_constants_useIX/OMEGA_2_TAU/MATLAB Function ==
  data: w1 input; T output; w2 input; w3 input; w4 input; k input
function T = fcn(w1, w2, w3, w4, k)

T = k*(w1^2 + w2^2 + w3^2 + w4^2);

== matlab function playground/ST_constants_useIX/OMEGA_2_TAU/MATLAB Function1 ==
  data: w2 input; tau_phi output; w4 input; kl input
function tau_phi = fcn(w2, w4, kl)

tau_phi = kl*(-w2^2 + w4^2);

== matlab function playground/ST_constants_useIX/OMEGA_2_TAU/MATLAB Function2 ==
  data: w1 input; tau_theta output; w3 input; kl input
function tau_theta = fcn(w1, w3, kl)

tau_theta = kl* (-w1^2 + w3^2);

== matlab function playground/ST_constants_useIX/OMEGA_2_TAU/MATLAB Function3 ==
  data: w1 input; tau_psi output; w2 input; w3 input; w4 input; b input
function tau_psi = fcn(w1, w2, w3, w4, b)

tau_psi = b * (-w1^2 + w2^2 - w3^2 + w4^2);
%tau_psi = b * (w1^2 - w2^2 + w3^2 - w4^2);

%tau_psi = b * (w1 - w2 + w3 - w4);

== matlab function playground/ST_constants_useIX/TAU_2_OMEGA/MATLAB Function1 ==
  data: T input; omega_1 output; omega_2 output; omega_3 output; omega_4 output; tau_phi input; tau_theta input; tau_psi input; k input; l input; b input
function [omega_1,omega_2,omega_3,omega_4] = fcn(T,tau_phi,tau_theta,tau_psi,k,l,b)
%omega_1 = tau_y/(4*k) + tau_theta/(2*k*l) + tau_psi/(4*b);
%omega_2 = tau_y/(4*k) + tau_gamma/(2*k*l) - tau_psi/(4*b);
%omega_3 = tau_y/(4*k) - tau_theta/(2*k*l) + tau_psi/(4*b);  % измененные по решению системы уравнений
%omega_4 = tau_y/(4*k) - tau_gamma/(2*k*l) - tau_psi/(4*b);

omega_1 = T/(4*k) - tau_theta/(2*k*l) - tau_psi/(4*b);
omega_2 = T/(4*k) - tau_phi/(2*k*l) + tau_psi/(4*b);  % согласно статье
omega_3 = T/(4*k) + tau_theta/(2*k*l) - tau_psi/(4*b);
omega_4 = T/(4*k) + tau_phi/(2*k*l) + tau_psi/(4*b);

== matlab function playground/ST_constants_useIX/XYZ POSITION/XYZ ==
  data: T input; ddx output; m input; Ax input; Ay input; Az input; phi input; theta input; psi input; dx input; dy input; dz input; ddy output; ddz output
function [ddx, ddy, ddz] = fcn(T, m, Ax, Ay, Az, phi, theta, psi, dx, dy, dz)

g = 9.81;

ddx = (T/m)*(cos(psi)*sin(theta)*cos(phi) + sin(psi)*sin(phi)) - Ax*dx/m;
ddy = (T/m)*(sin(psi)*sin(theta)*cos(phi) - cos(psi)*sin(phi)) - Ay*dy/m;

ddz = -g + (T/m)*(cos(theta)*cos(phi)) - Az*dz/m;

== matlab function playground/ST_constants_no_IX/ANGLS/psi_part ==
  data: q input; d_psi output; r input; phi input; theta input
function d_psi = fcn(q, r, phi, theta)

d_psi = q*sin(phi)/cos(theta) + r*cos(phi)/cos(theta);

== matlab function playground/ST_constants_no_IX/ANGLS/theta_part ==
  data: q input; d_theta output; r input; phi input
function d_theta = fcn(q, r, phi)

d_theta = cos(phi)*q - sin(phi)*r;
